simulink model "hld_ofdm_rx"  (R2017b)
settings: Solver=VariableStepAuto  StartTime=0.0  StopTime=10.0  RelTol=1e-3
libraries: commdigbbndam3 x16, hdlsllib x2, dspxfrm3 x1
settings Model: Creator=jake  LastModifiedBy=mw
settings CodeAppCC: StateflowObjectComments=on

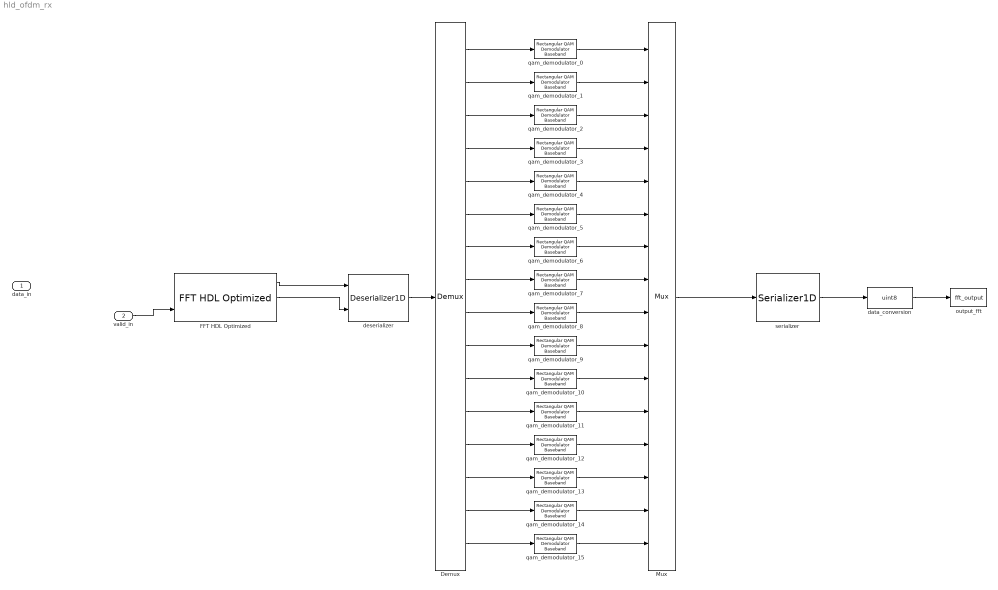
== system hld_ofdm_rx ==
  data_in : Inport  OutDataTypeStr=fixdt(1,37,27)
  valid_in : Inport  Port=2  OutDataTypeStr=fixdt(1,37,27)
  Demux : Demux  Outputs=16
  FFT HDL Optimized : dspxfrm3/FFT HDL Optimized  FFTLength=16  Architecture=Burst Radix 2  ComplexMultiplication=Use 3 multipliers and 5 adders  BitReversedOutput=on  BitReversedInput=off  Normalize=off  SimulateUsing=Code generation  RoundingMethod=Floor  ResetInputPort=off  StartOutputPort=off  EndOutputPort=off
      settings: SourceProductName=DSP System Toolbox  SourceProductBaseCode=DS
  Mux : Mux  Inputs=16
  data_conversion : DataTypeConversion  OutDataTypeStr=uint8
  deserializer : hdlsllib/HDL Operations/Deserializer1D  Ratio=16  IdleCycles=0  InitialCondition=0  startIn=off  validIn=on  validOut=off  inputDataDimensions=-1  inputSampleTime=-1  inputSignalType=auto
      settings: SourceProductName=HDL Coder  SourceProductBaseCode=HD
  output_fft : ToWorkspace  VariableName=fft_output  SampleTime=-1
  qam_demodulator_{0..15} (16 alike) : commdigbbndam3/Rectangular QAM Demodulator Baseband  M=16  OutType=Integer  DecType=Hard decision  VarSource=Dialog  Variance=1  Dec=Gray  Mapping=[0:15]  PowType=Min. distance between symbols  MinDist=2  AvgPow=1  PeakPow=1  Ph=0  outDtype1=Inherit via internal rule  outDtype2=Inherit via internal rule  derotateFactorWordLen=16  derotateFactorDataTypeStr=Inherit: Same word length as input  derotateFactorLastDataTypeStr=Inherit: Same word length as input  denormFactorWordLen=16  denormFactorDataTypeStr=Inherit: Same word length as input  denormFactorLastDataTypeStr=Inherit: Same word length as input  prodOutWordLen=32  prodOutOverflowMode=Wrap  prodOutRoundingMode=Floor  prodOutOvFlMode=off  prodOutOvFlModeLastStrValue=off  sumWordLen=32
  serializer : hdlsllib/HDL Operations/Serializer1D  Ratio=16  IdleCycles=0  validIn=off  startOut=off  validOut=off  inputDataDimensions=-1  inputSampleTime=-1  inputSignalType=auto
      settings: SourceProductName=HDL Coder  SourceProductBaseCode=HD
  wires:
  Demux/1 -> qam_demodulator_0/1
  Demux/2 -> qam_demodulator_1/1
  Demux/3 -> qam_demodulator_2/1
  Demux/4 -> qam_demodulator_3/1
  Demux/5 -> qam_demodulator_4/1
  Demux/6 -> qam_demodulator_5/1
  Demux/7 -> qam_demodulator_6/1
  Demux/8 -> qam_demodulator_7/1
  Demux/9 -> qam_demodulator_8/1
  Demux/10 -> qam_demodulator_9/1
  Demux/11 -> qam_demodulator_10/1
  Demux/12 -> qam_demodulator_11/1
  Demux/13 -> qam_demodulator_12/1
  Demux/14 -> qam_demodulator_13/1
  Demux/15 -> qam_demodulator_14/1
  Demux/16 -> qam_demodulator_15/1
  qam_demodulator_0/1 -> Mux/1
  qam_demodulator_1/1 -> Mux/2
  qam_demodulator_2/1 -> Mux/3
  qam_demodulator_3/1 -> Mux/4
  qam_demodulator_4/1 -> Mux/5
  qam_demodulator_5/1 -> Mux/6
  qam_demodulator_6/1 -> Mux/7
  qam_demodulator_7/1 -> Mux/8
  qam_demodulator_8/1 -> Mux/9
  qam_demodulator_9/1 -> Mux/10
  qam_demodulator_10/1 -> Mux/11
  qam_demodulator_11/1 -> Mux/12
  qam_demodulator_12/1 -> Mux/13
  qam_demodulator_13/1 -> Mux/14
  qam_demodulator_14/1 -> Mux/15
  qam_demodulator_15/1 -> Mux/16
  Mux/1 -> serializer/1
  serializer/1 -> data_conversion/1
  data_conversion/1 -> output_fft/1
  FFT HDL Optimized/1 -> deserializer/1
  deserializer/1 -> Demux/1
  FFT HDL Optimized/2 -> deserializer/2
  valid_in/1 -> FFT HDL Optimized/2
